simulink model "exercise03_simulation_model_solution_part1"  (R2025b)
settings: Solver=ode45  StartTime=0.0  StopTime=10  FixedStep=1e-5  MaxStep=1e-3  RelTol=1e-4  EnableMultiTasking=on
PreLoadFcn:
  | exercise03_simulation_parameters
values from neighbouring files (symbols this model uses):
  g = 9.81    [exercise03_solution_compute_LQR_outer_loop_controller.m]
undefined symbols (not defined in the file or in its folder): cmd_2_newtons_conversion_linear_coefficient, cmd_2_newtons_conversion_quadratic_coefficient, cmd_max, cmd_min, DiscIntNeverNeededParam, K_lqr, measurement_noise, nrotor_initial_conditions, nrotor_vehicle, pid_x, pid_y, pid_z, reference, sample_time, sigbuilder_block
libraries: simulink x3
(part 1 of 2)
settings Model: Creator=kimal and jseitz  LastModifiedBy=resjoehr
settings SolverCC: ZeroCrossControl=DisableAll  AlgebraicLoopSolver=TrustRegion  AutoInsertRateTranBlk=on
settings DataIOCC: LimitDataPoints=on  SaveFormat=Array  ReturnWorkspaceOutputs=off
settings OptimizationCC: LifeSpan=inf
settings DebuggingCC: SolverPrmCheckMsg=warning  UnconnectedInputMsg=warning  UnconnectedOutputMsg=warning  UnconnectedLineMsg=warning  SFUnexpectedBacktrackingDiag=warning  SFNoUnconditionalDefaultTransitionDiag=warning  SFExecutionAtInitializationDiag=none  ArithmeticOperatorsInVariantConditions=warning
settings HardwareCC: ProdBitPerPointer=32.0  ProdBitPerSizeT=32.0  ProdBitPerPtrDiffT=32.0  ProdLargestAtomicFloat=None  ProdIntDivRoundTo=Undefined  ProdEndianess=Unspecified  ProdWordSize=32.0  ProdHWDeviceType=32-bit Generic
settings ModelReferenceCC: EnableRefExpFcnMdlSchedulingChecks=on  PropagateSignalLabelsOutOfModel=off
settings SFSimCC: SimUseLocalCustomCode=off  CustomCodeUndefinedFunction=UseInterfaceOnly
settings RTWCC: RTWUseLocalCustomCode=off  GPUComputeCapability=3.5
settings CodeAppCC: StateflowObjectComments=on
settings GRTTargetCC: TargetLangStandard=C89/C90 (ANSI)
settings ConfigComp: CovMetricSettings=dw  CovSaveCumulativeToWorkspaceVar=on  CovSaveSingleToWorkspaceVar=on  CovExternalEMLEnable=off  CovSFcnEnable=off
settings SimscapeCC: SimscapeNormalizeSystem=off
settings ConfigurationSet: Description=SimMechanics 2G

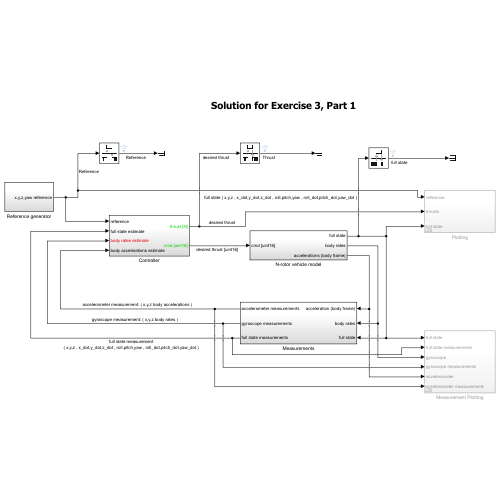
[thumbnail: Simulink's stored preview of the top-level diagram]
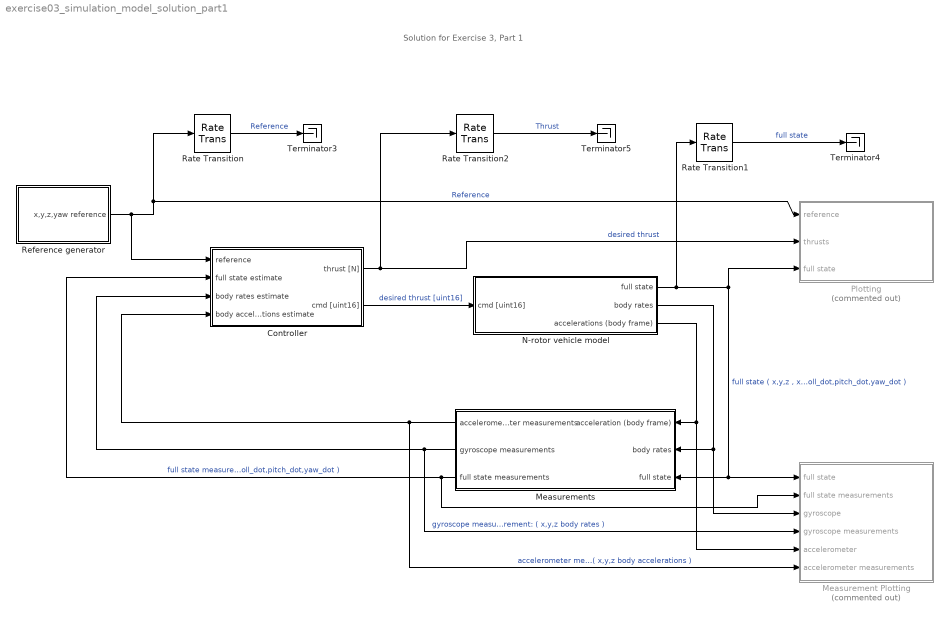
== system exercise03_simulation_model_solution_part1 ==
  note: Solution for Exercise 3, Part 1
  Controller : Subsystem
  Measurement Plotting : Subsystem  Commented=on
  Measurements : Subsystem
  N-rotor vehicle model : Subsystem
  Plotting : Subsystem  Commented=on
  Rate Transition : RateTransition  OutPortSampleTime=0.05
  Rate Transition1 : RateTransition  OutPortSampleTime=0.05
  Rate Transition2 : RateTransition  OutPortSampleTime=0.05
  Reference generator : Subsystem
  Terminator3 : Terminator
  Terminator4 : Terminator
  Terminator5 : Terminator
  wires:
  N-rotor vehicle model/2(body rates) -> Measurement Plotting/3(gyroscope), Measurements/2(body rates)
  N-rotor vehicle model/3(accelerations (body frame)) -> Measurement Plotting/5(accelerometer), Measurements/1(acceleration (body frame))
  Measurements/3(full state measurements) -> Controller/2(full state estimate), Measurement Plotting/2(full state measurements)  "full state measurement ( x,y,z , x_dot,y_dot,z_dot , roll,pitch,yaw , roll_dot,pitch_dot,yaw_dot )"
  Measurements/1(accelerometer measurements) -> Controller/4(body accelerations estimate), Measurement Plotting/6(accelerometer measurements)  "accelerometer measurement: ( x,y,z body accelerations )"
  Measurements/2(gyroscope measurements) -> Controller/3(body rates estimate), Measurement Plotting/4(gyroscope measurements)  "gyroscope measurement: ( x,y,z body rates )"
  Controller/2(cmd [uint16]) -> N-rotor vehicle model/1(cmd [uint16])  "desired thrust [uint16]"
  Reference generator/1(x,y,z,yaw reference) -> Controller/1(reference), Rate Transition/1, Plotting/1(reference)  "Reference"
  Rate Transition2/1 -> Terminator5/1  "Thrust"
  Rate Transition1/1 -> Terminator4/1  "full state"
  Controller/1(thrust [N]) -> Rate Transition2/1, Plotting/2(thrusts)  "desired thrust"
  Rate Transition/1 -> Terminator3/1  "Reference"
  N-rotor vehicle model/1(full state) -> Rate Transition1/1, Measurement Plotting/1(full state), Measurements/3(full state), Plotting/3(full state)  "full state ( x,y,z , x_dot,y_dot,z_dot , roll,pitch,yaw , roll_dot,pitch_dot,yaw_dot )"

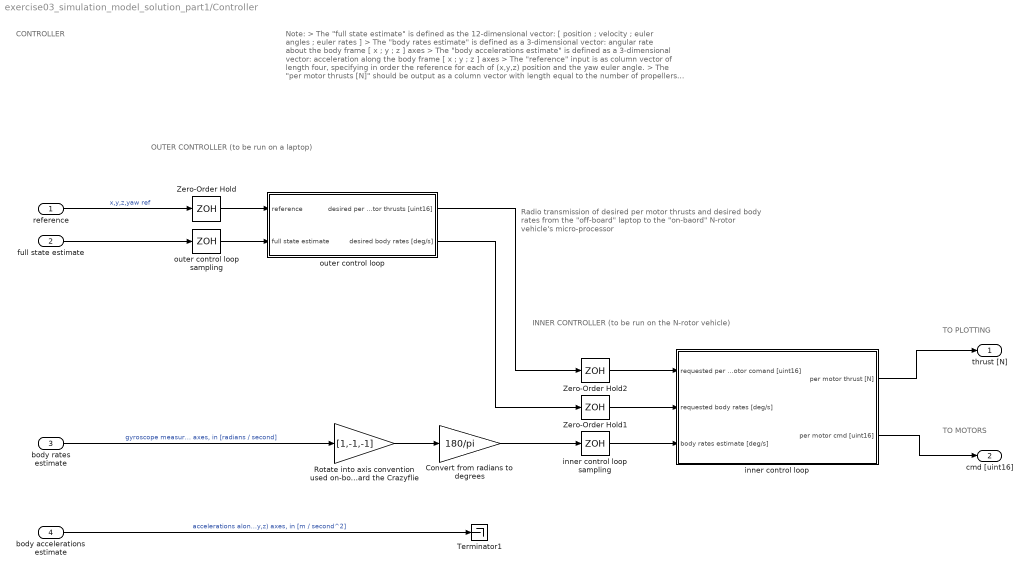
== system exercise03_simulation_model_solution_part1/Controller ==
  note: CONTROLLER
  note: Note:
      | > The "full state estimate" is defined as the 12-dimensional vector: [ position ; velocity ; euler angles ; euler rates ]
      | > The "body rates estimate" is defined as a 3-dimensional vector: angular rate about the body frame [ x ; y ; z ] axes
      | > The "body accelerations estimate" is defined as a 3-dimensional vector: acceleration along the body frame [ x ; y ; z ] axes
      | > The "reference" input is as column vector of length four, specifying in order the reference for each of (x,y,z) position and the yaw euler angle.
      | > The "per motor thrusts [N]" should be output as a column vector with length equal to the number of propellers on the vehicle, i.e., with length equal to N
      | > The "per motor cmd [uint16]" should be output as a column vector with length equal to the number of propellers on the vehicle, i.e., with length equal to N
  note: TO PLOTTING
  note: TO MOTORS
  note: Radio transmission of desired
      | per motor thrusts and desired
      | body rates from the "off-board"
      | laptop to the "on-baord" N-rotor
      | vehicle's micro-processor
  note: OUTER CONTROLLER (to be run on a laptop)
  note: INNER CONTROLLER (to be run on the N-rotor vehicle)
  reference : Inport
  full state estimate : Inport  Port=2
  body rates estimate : Inport  Port=3
  body accelerations estimate : Inport  Port=4
  Convert from radians to degrees : Gain  Gain=180/pi
  Rotate into axis convention used on-board the Crazyflie : Gain  Gain=[1,-1,-1]
  Terminator1 : Terminator
  Zero-Order Hold : ZeroOrderHold  SampleTime=sample_time.controller_outer
  Zero-Order Hold1 : ZeroOrderHold  SampleTime=sample_time.controller_inner
  Zero-Order Hold2 : ZeroOrderHold  SampleTime=sample_time.controller_inner
  inner control loop sampling : ZeroOrderHold  SampleTime=sample_time.controller_inner
  inner control loop : Subsystem
  outer control loop sampling : ZeroOrderHold  SampleTime=sample_time.controller_outer
  outer control loop : Subsystem
  thrust [N] : Outport  VectorParamsAs1DForOutWhenUnconnected=off
  cmd [uint16] : Outport  Port=2  VectorParamsAs1DForOutWhenUnconnected=off
  wires:
  body accelerations estimate/1 -> Terminator1/1  "accelerations along the body frame (x,y,z) axes, in [m / second^2]"
  body rates estimate/1 -> Rotate into axis convention used on-board the Crazyflie/1  "gyroscope measurement: angular rates about the body frame (x,y,z) axes, in [radians / second]"
  inner control loop/1(per motor thrust [N]) -> thrust [N]/1
  reference/1 -> Zero-Order Hold/1  "x,y,z,yaw ref"
  inner control loop/2(per motor cmd [uint16]) -> cmd [uint16]/1
  outer control loop sampling/1 -> outer control loop/2(full state estimate)
  full state estimate/1 -> outer control loop sampling/1
  outer control loop/2(desired body rates [deg/s]) -> Zero-Order Hold1/1
  Rotate into axis convention used on-board the Crazyflie/1 -> Convert from radians to degrees/1
  outer control loop/1(desired per motor thrusts [uint16]) -> Zero-Order Hold2/1
  Convert from radians to degrees/1 -> inner control loop sampling/1
  Zero-Order Hold1/1 -> inner control loop/2(requested body rates [deg/s])
  Zero-Order Hold/1 -> outer control loop/1(reference)
  Zero-Order Hold2/1 -> inner control loop/1(requested per motor comand [uint16])
  inner control loop sampling/1 -> inner control loop/3(body rates estimate [deg/s])

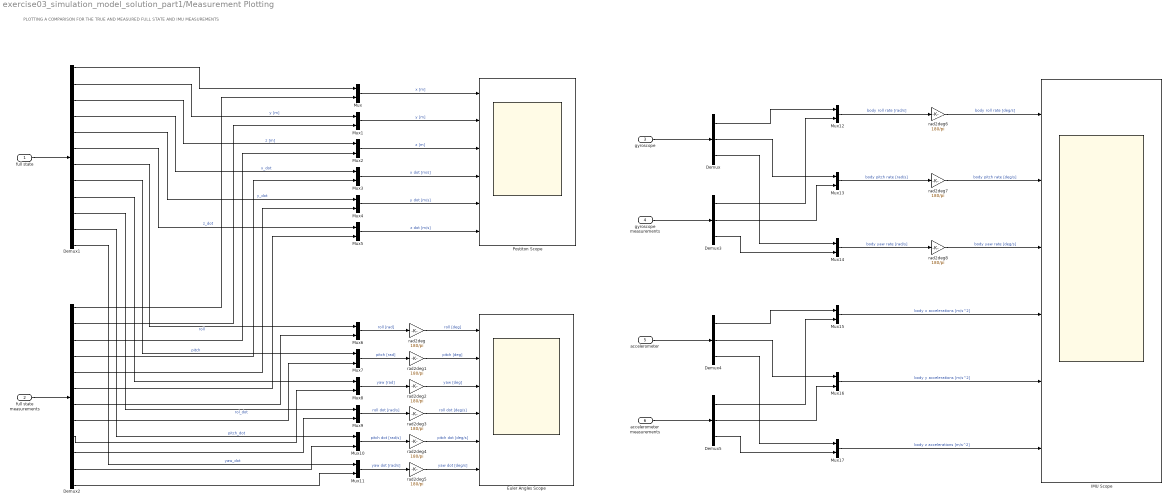
== system exercise03_simulation_model_solution_part1/Measurement Plotting ==
  note: PLOTTING A COMPARISON FOR THE TRUE AND MEASURED FULL STATE AND IMU MEASUREMENTS
  full state : Inport
  full state measurements : Inport  Port=2
  gyroscope : Inport  Port=3
  gyroscope measurements : Inport  Port=4
  accelerometer : Inport  Port=5
  accelerometer measurements : Inport  Port=6
  Demux{,3..5} (4 alike) : Demux  Outputs=3
  Demux1 : Demux  Outputs=12
  Demux2 : Demux  Outputs=12
  Euler Angles Scope : Scope  NumInputPorts=6
      settings: TimeSpan=10  ActiveDisplayYMinimum=-7.01847  ActiveDisplayYMaximum=5.9111  DataLoggingSaveFormat=Array
  IMU Scope : Scope  NumInputPorts=6
      settings: TimeSpan=10  ActiveDisplayYMinimum=-766.14622  ActiveDisplayYMaximum=735.9979  DataLoggingSaveFormat=Array
  Mux{,1..17} (18 alike) : Mux  Inputs=2
  Postiton Scope : Scope  NumInputPorts=6
      settings: TimeSpan=10  ActiveDisplayYMinimum=-0.0967  ActiveDisplayYMaximum=0.63434  DataLoggingSaveFormat=Array
  rad2deg{,1..8} (9 alike) : Gain  Gain=180/pi
  wires:
  full state/1 -> Demux1/1
  full state measurements/1 -> Demux2/1
  Mux/1 -> Postiton Scope/1  "x [m]"
  Mux1/1 -> Postiton Scope/2  "y [m]"
  Mux2/1 -> Postiton Scope/3  "z [m]"
  Mux3/1 -> Postiton Scope/4  "x dot [m/s]"
  Mux4/1 -> Postiton Scope/5  "y dot [m/s]"
  Mux5/1 -> Postiton Scope/6  "z dot [m/s]"
  Mux6/1 -> rad2deg/1  "roll [rad]"
  Mux7/1 -> rad2deg1/1  "pitch [rad]"
  Mux8/1 -> rad2deg2/1  "yaw [rad]"
  Mux9/1 -> rad2deg3/1  "roll dot [rad/s]"
  Mux10/1 -> rad2deg4/1  "pitch dot [rad/s]"
  Mux11/1 -> rad2deg5/1  "yaw dot [rad/s]"
  rad2deg/1 -> Euler Angles Scope/1  "roll [deg]"
  rad2deg2/1 -> Euler Angles Scope/3  "yaw [deg]"
  rad2deg1/1 -> Euler Angles Scope/2  "pitch [deg]"
  rad2deg3/1 -> Euler Angles Scope/4  "roll dot [deg/s]"
  rad2deg4/1 -> Euler Angles Scope/5  "pitch dot [deg/s]"
  rad2deg5/1 -> Euler Angles Scope/6  "yaw dot [deg/s]"
  Demux1/1 -> Mux/1
  Demux2/1 -> Mux/2
  Demux1/2 -> Mux1/1  "y [m]"
  Demux1/3 -> Mux2/1  "z [m]"
  Demux2/2 -> Mux1/2
  Demux2/3 -> Mux2/2
  Demux1/4 -> Mux3/1  "x_dot"
  Demux1/5 -> Mux4/1  "y_dot"
  Demux1/6 -> Mux5/1  "z_dot"
  Demux1/12 -> Mux11/1  "yaw_dot"
  Demux1/11 -> Mux10/1  "pitch_dot"
  Demux1/10 -> Mux9/1  "rol_dot"
  Demux1/9 -> Mux8/1
  Demux1/8 -> Mux7/1  "pitch"
  Demux1/7 -> Mux6/1  "roll"
  Demux2/4 -> Mux3/2
  Demux2/5 -> Mux4/2
  Demux2/6 -> Mux5/2
  Demux2/7 -> Mux6/2
  Demux2/8 -> Mux7/2
  Demux2/9 -> Mux8/2
  Demux2/10 -> Mux9/2
  Demux2/11 -> Mux10/2
  Demux2/12 -> Mux11/2
  gyroscope measurements/1 -> Demux3/1
  gyroscope/1 -> Demux/1
  Mux12/1 -> rad2deg6/1  "body roll rate [rad/s]"
  rad2deg6/1 -> IMU Scope/1  "body roll rate [deg/s]"
  Mux13/1 -> rad2deg7/1  "body pitch rate [rad/s]"
  rad2deg7/1 -> IMU Scope/2  "body pitch rate [deg/s]"
  Mux14/1 -> rad2deg8/1  "body yaw rate [rad/s]"
  rad2deg8/1 -> IMU Scope/3  "body yaw rate [deg/s]"
  Demux/1 -> Mux12/1
  Demux/2 -> Mux13/1
  Demux/3 -> Mux14/1
  Demux3/3 -> Mux14/2
  Demux3/2 -> Mux13/2
  Demux3/1 -> Mux12/2
  accelerometer measurements/1 -> Demux5/1
  accelerometer/1 -> Demux4/1
  Mux15/1 -> IMU Scope/4  "body x accelerations [m/s^2]"
  Mux16/1 -> IMU Scope/5  "body y accelerations [m/s^2]"
  Mux17/1 -> IMU Scope/6  "body z accelerations [m/s^2]"
  Demux4/1 -> Mux15/1
  Demux4/2 -> Mux16/1
  Demux4/3 -> Mux17/1
  Demux5/3 -> Mux17/2
  Demux5/2 -> Mux16/2
  Demux5/1 -> Mux15/2

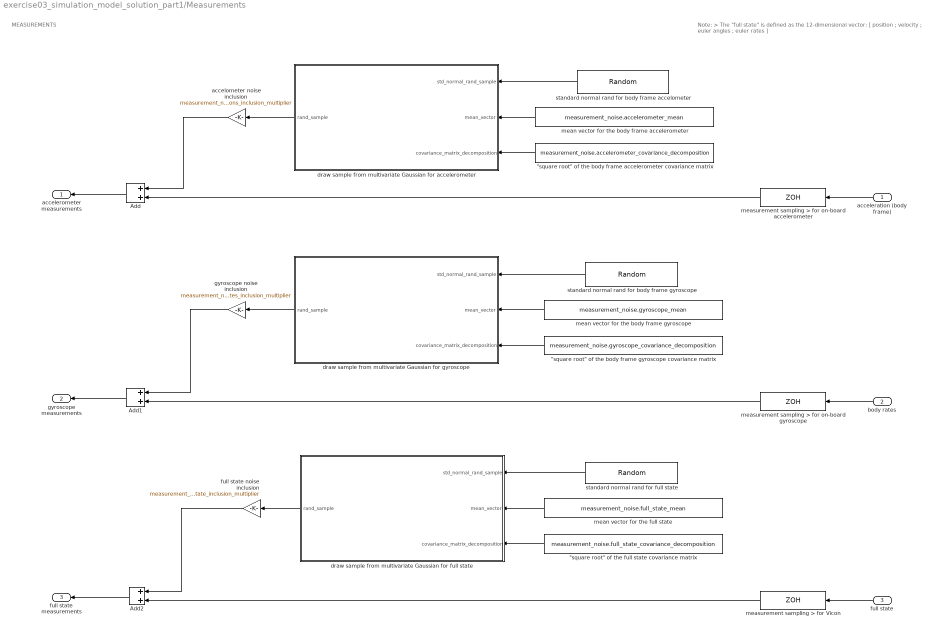
== system exercise03_simulation_model_solution_part1/Measurements ==
  note: Note:
      | > The "full state" is defined as the 12-dimensional vector:
      | [ position ; velocity ; euler angles ; euler rates ]
  note: MEASUREMENTS
  acceleration (body frame) : Inport
  body rates : Inport  Port=2
  full state : Inport  Port=3
  "\"square root\" of the body frame accelerometer covariance matrix" : Constant  Value=measurement_noise.accelerometer_covariance_decomposition
  "\"square root\" of the body frame gyroscope covariance matrix" : Constant  Value=measurement_noise.gyroscope_covariance_decomposition
  "\"square root\" of the full state covariance matrix" : Constant  Value=measurement_noise.full_state_covariance_decomposition
  Add : Sum
  Add1 : Sum
  Add2 : Sum
  accelometer noise inclusion : Gain  Gain=measurement_noise.body_accelerations_inclusion_multiplier
  draw sample from multivariate Gaussian for accelerometer : MATLAB Function  TreatAsAtomicUnit=on
  draw sample from multivariate Gaussian for full state : MATLAB Function  TreatAsAtomicUnit=on
  draw sample from multivariate Gaussian for gyroscope : MATLAB Function  TreatAsAtomicUnit=on
  full state noise inclusion : Gain  Gain=measurement_noise.full_state_inclusion_multiplier
  gyroscope noise inclusion : Gain  Gain=measurement_noise.body_rates_inclusion_multiplier
  mean vector for the body frame accelerometer : Constant  Value=measurement_noise.accelerometer_mean
  mean vector for the body frame gyroscope : Constant  Value=measurement_noise.gyroscope_mean
  mean vector for the full state : Constant  Value=measurement_noise.full_state_mean
  measurement sampling > for Vicon : ZeroOrderHold  SampleTime=sample_time.measurements_full_state
  measurement sampling > for on-board accelerometer : ZeroOrderHold  SampleTime=sample_time.measurements_body_accelerations
  measurement sampling > for on-board gyroscope : ZeroOrderHold  SampleTime=sample_time.measurements_body_rates
  standard normal rand for body frame accelometer : RandomNumber  Mean=measurement_noise.accelerometer_mean  Variance=measurement_noise.accelerometer_var  Seed=measurement_noise.accelerometer_seed  SampleTime=sample_time.measurements_body_accelerations  VectorParams1D=off
  standard normal rand for body frame gyroscope : RandomNumber  Mean=measurement_noise.gyroscope_mean  Variance=measurement_noise.gyroscope_var  Seed=measurement_noise.gyroscope_seed  SampleTime=sample_time.measurements_body_rates  VectorParams1D=off
  standard normal rand for full state : RandomNumber  Mean=zeros(12,1)  Variance=ones(12,1)  Seed=measurement_noise.full_state_seed  SampleTime=sample_time.measurements_full_state  VectorParams1D=off
  accelerometer measurements : Outport  VectorParamsAs1DForOutWhenUnconnected=off
  gyroscope measurements : Outport  Port=2  VectorParamsAs1DForOutWhenUnconnected=off
  full state measurements : Outport  Port=3  VectorParamsAs1DForOutWhenUnconnected=off
  wires:
  full state/1 -> measurement sampling > for Vicon/1
  acceleration (body frame)/1 -> measurement sampling > for on-board accelerometer/1
  body rates/1 -> measurement sampling > for on-board gyroscope/1
  measurement sampling > for Vicon/1 -> Add2/2
  "\"square root\" of the full state covariance matrix"/1 -> draw sample from multivariate Gaussian for full state/3(covariance_matrix_decomposition)
  mean vector for the full state/1 -> draw sample from multivariate Gaussian for full state/2(mean_vector)
  mean vector for the body frame gyroscope/1 -> draw sample from multivariate Gaussian for gyroscope/2(mean_vector)
  gyroscope noise inclusion/1 -> Add1/1
  measurement sampling > for on-board accelerometer/1 -> Add/2
  mean vector for the body frame accelerometer/1 -> draw sample from multivariate Gaussian for accelerometer/2(mean_vector)
  draw sample from multivariate Gaussian for accelerometer/1(rand_sample) -> accelometer noise inclusion/1
  draw sample from multivariate Gaussian for gyroscope/1(rand_sample) -> gyroscope noise inclusion/1
  standard normal rand for full state/1 -> draw sample from multivariate Gaussian for full state/1(std_normal_rand_sample)
  "\"square root\" of the body frame gyroscope covariance matrix"/1 -> draw sample from multivariate Gaussian for gyroscope/3(covariance_matrix_decomposition)
  accelometer noise inclusion/1 -> Add/1
  draw sample from multivariate Gaussian for full state/1(rand_sample) -> full state noise inclusion/1
  full state noise inclusion/1 -> Add2/1
  measurement sampling > for on-board gyroscope/1 -> Add1/2
  standard normal rand for body frame gyroscope/1 -> draw sample from multivariate Gaussian for gyroscope/1(std_normal_rand_sample)
  standard normal rand for body frame accelometer/1 -> draw sample from multivariate Gaussian for accelerometer/1(std_normal_rand_sample)
  Add2/1 -> full state measurements/1
  "\"square root\" of the body frame accelerometer covariance matrix"/1 -> draw sample from multivariate Gaussian for accelerometer/3(covariance_matrix_decomposition)
  Add/1 -> accelerometer measurements/1
  Add1/1 -> gyroscope measurements/1

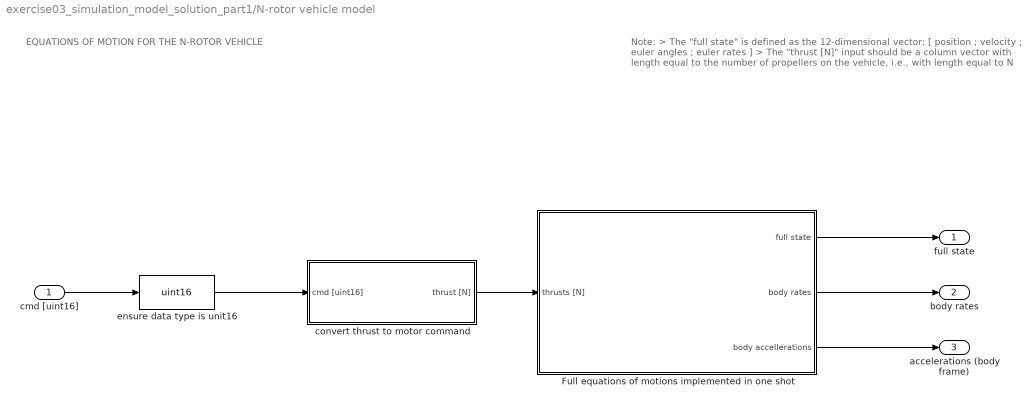
== system exercise03_simulation_model_solution_part1/N-rotor vehicle model ==
  note: Note:
      | > The "full state" is defined as the 12-dimensional vector:
      | [ position ; velocity ; euler angles ; euler rates ]
      | > The "thrust [N]" input should be a column vector with
      | length equal to the number of propellers on the vehicle,
      | i.e., with length equal to N
  note: EQUATIONS OF MOTION FOR THE N-ROTOR VEHICLE
  cmd [uint16] : Inport
  Full equations of motions implemented in one shot : Subsystem
  convert thrust to motor command : Subsystem
  ensure data type is unit16 : DataTypeConversion  OutDataTypeStr=uint16  SaturateOnIntegerOverflow=off  RndMeth=Floor
  full state : Outport  VectorParamsAs1DForOutWhenUnconnected=off
  body rates : Outport  Port=2  VectorParamsAs1DForOutWhenUnconnected=off
  accelerations (body frame) : Outport  Port=3  VectorParamsAs1DForOutWhenUnconnected=off
  wires:
  cmd [uint16]/1 -> ensure data type is unit16/1
  Full equations of motions implemented in one shot/1(full state) -> full state/1
  Full equations of motions implemented in one shot/2(body rates) -> body rates/1
  Full equations of motions implemented in one shot/3(body accellerations) -> accelerations (body frame)/1
  convert thrust to motor command/1(thrust [N]) -> Full equations of motions implemented in one shot/1(thrusts [N])
  ensure data type is unit16/1 -> convert thrust to motor command/1(cmd [uint16])

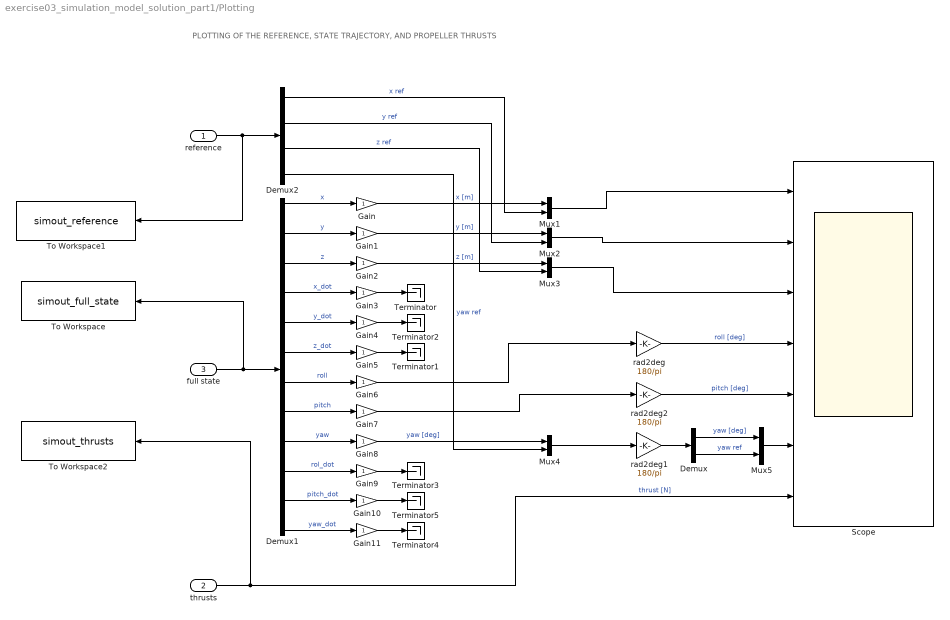
== system exercise03_simulation_model_solution_part1/Plotting ==
  note: PLOTTING OF THE REFERENCE, STATE TRAJECTORY, AND PROPELLER THRUSTS
  reference : Inport
  thrusts : Inport  Port=2
  full state : Inport  Port=3
  Demux : Demux  Outputs=2
  Demux1 : Demux  Outputs=12
  Demux2 : Demux
  Gain{,1..11} (12 alike) : Gain
  Mux{1..5} (5 alike) : Mux  Inputs=2
  Scope : Scope  NumInputPorts=7
      settings: TimeSpan=10  ActiveDisplayYMinimum=-1.3075  ActiveDisplayYMaximum=11.45582  DataLoggingSaveFormat=Array
  Terminator{,1..5} (6 alike) : Terminator
  To Workspace : ToWorkspace  VariableName=simout_full_state  SaveFormat=Timeseries  SampleTime=-1
  To Workspace1 : ToWorkspace  VariableName=simout_reference  SaveFormat=Timeseries  SampleTime=-1
  To Workspace2 : ToWorkspace  VariableName=simout_thrusts  SaveFormat=Timeseries  SampleTime=-1
  rad2deg : Gain  Gain=180/pi
  rad2deg1 : Gain  Gain=180/pi
  rad2deg2 : Gain  Gain=180/pi
  wires:
  Demux1/1 -> Gain/1  "x"
  Demux1/2 -> Gain1/1  "y"
  Demux1/6 -> Gain5/1  "z_dot"
  Gain7/1 -> rad2deg2/1
  Demux1/8 -> Gain7/1  "pitch"
  full state/1 -> To Workspace/1, Demux1/1
  Demux1/5 -> Gain4/1  "y_dot"
  Demux1/7 -> Gain6/1  "roll"
  Demux1/4 -> Gain3/1  "x_dot"
  Demux1/3 -> Gain2/1  "z"
  Gain6/1 -> rad2deg/1
  Demux1/9 -> Gain8/1  "yaw"
  Demux1/10 -> Gain9/1  "rol_dot"
  Demux1/11 -> Gain10/1  "pitch_dot"
  Demux1/12 -> Gain11/1  "yaw_dot"
  Gain9/1 -> Terminator3/1
  Gain10/1 -> Terminator5/1
  Gain11/1 -> Terminator4/1
  Gain3/1 -> Terminator/1
  Gain4/1 -> Terminator2/1
  Gain5/1 -> Terminator1/1
  thrusts/1 -> To Workspace2/1, Scope/7  "thrust [N]"
  reference/1 -> To Workspace1/1, Demux2/1
  Mux1/1 -> Scope/1
  Mux2/1 -> Scope/2
  Gain/1 -> Mux1/1  "x [m]"
  Demux2/1 -> Mux1/2  "x ref"
  Gain1/1 -> Mux2/1  "y [m]"
  Demux2/2 -> Mux2/2  "y ref"
  Mux3/1 -> Scope/3
  Gain2/1 -> Mux3/1  "z [m]"
  Demux2/3 -> Mux3/2  "z ref"
  Mux4/1 -> rad2deg1/1
  Gain8/1 -> Mux4/1  "yaw [deg]"
  Demux2/4 -> Mux4/2  "yaw ref"
  rad2deg/1 -> Scope/4  "roll [deg]"
  rad2deg2/1 -> Scope/5  "pitch [deg]"
  Demux/1 -> Mux5/1  "yaw [deg]"
  Demux/2 -> Mux5/2  "yaw ref"
  rad2deg1/1 -> Demux/1
  Mux5/1 -> Scope/6

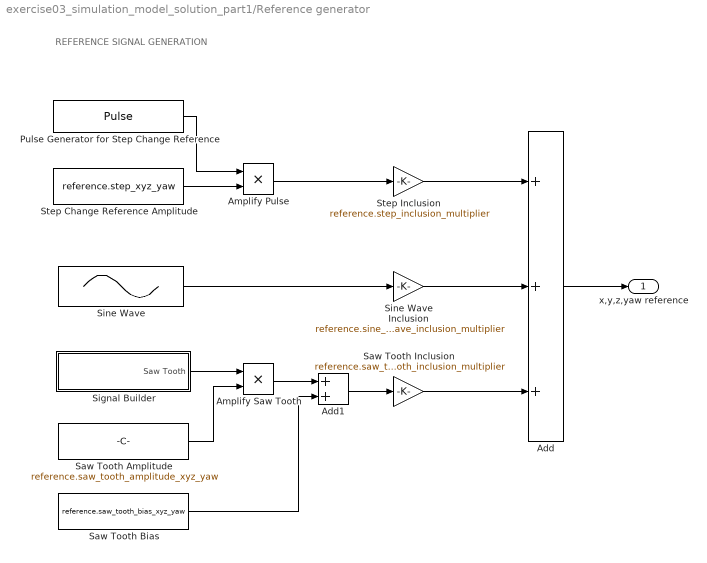
== system exercise03_simulation_model_solution_part1/Reference generator ==
  note: REFERENCE SIGNAL GENERATION
  Add : Sum  Inputs=+++
  Add1 : Sum
  Amplify Pulse : Product
  Amplify Saw Tooth : Product
  Pulse Generator for Step Change Reference : DiscretePulseGenerator  PulseType=Time based  Period=reference.step_period*2  PulseWidth=50
  Saw Tooth Amplitude : Constant  Value=reference.saw_tooth_amplitude_xyz_yaw
  Saw Tooth Bias : Constant  Value=reference.saw_tooth_bias_xyz_yaw
  Saw Tooth Inclusion : Gain  Gain=reference.saw_tooth_inclusion_multiplier
  Signal Builder : Subsystem  Tag=STV Subsys  LoadFcn=sigbuilder_block('load');  StartFcn=sigbuilder_block('start');  StopFcn=sigbuilder_block('stop');  ClipboardFcn=sigbuilder_block('clipboard');  mask(Sigbuilder block){tuvar=[0:10]}
      mask help: Simulink:masks:SigbuilderBlock_MD
      mask init:
      | if ~strcmp(get_param(bdroot(gcbh),'SimulationStatus'),'stopped') tuvar = sigbuilder_block('maskInit'); end
      settings: CopyFcn=sigbuilder_block('copy');  DeleteFcn=sigbuilder_block('delete');  ModelCloseFcn=sigbuilder_block('modelClose');  PreSaveFcn=sigbuilder_block('preSave');  PauseFcn=sigbuilder_block('pause');  ContinueFcn=sigbuilder_block('continue');  NameChangeFcn=sigbuilder_block('namechange');  OpenFcn=sigbuilder_block('open',[-1646.25 158.25 895.5 539.25 ]);  CloseFcn=sigbuilder_block('close');
      mask Display: plot(0, 0, 100, 100,[2, 2, 32, 32, 2], [68, 8, 8, 68, 68],[32, 2], [38, 38], [32, 19, 2],[53, 60, 44], [32, 17, 17, 2],[16, 16, 31, 31]);txt = getActiveGroup(gcbh);text(2, 100, txt,'verticalAlignment', 'top');
  Sine Wave : Sin  Amplitude=reference.sine_amplitude_xyz_yaw  Bias=reference.sine_bias_xyz_yaw  Frequency=2*pi()/reference.sine_period  SampleTime=0
  Sine Wave Inclusion : Gain  Gain=reference.sine_wave_inclusion_multiplier
  Step Change Reference Amplitude : Constant  Value=reference.step_xyz_yaw
  Step Inclusion : Gain  Gain=reference.step_inclusion_multiplier
  x,y,z,yaw reference : Outport  VectorParamsAs1DForOutWhenUnconnected=off
  wires:
  Step Change Reference Amplitude/1 -> Amplify Pulse/2
  Pulse Generator for Step Change Reference/1 -> Amplify Pulse/1
  Sine Wave/1 -> Sine Wave Inclusion/1
  Add/1 -> x,y,z,yaw reference/1
  Step Inclusion/1 -> Add/1
  Sine Wave Inclusion/1 -> Add/2
  Amplify Pulse/1 -> Step Inclusion/1
  Saw Tooth Inclusion/1 -> Add/3
  Signal Builder/1(Saw Tooth) -> Amplify Saw Tooth/1
  Saw Tooth Amplitude/1 -> Amplify Saw Tooth/2
  Amplify Saw Tooth/1 -> Add1/1
  Add1/1 -> Saw Tooth Inclusion/1
  Saw Tooth Bias/1 -> Add1/2

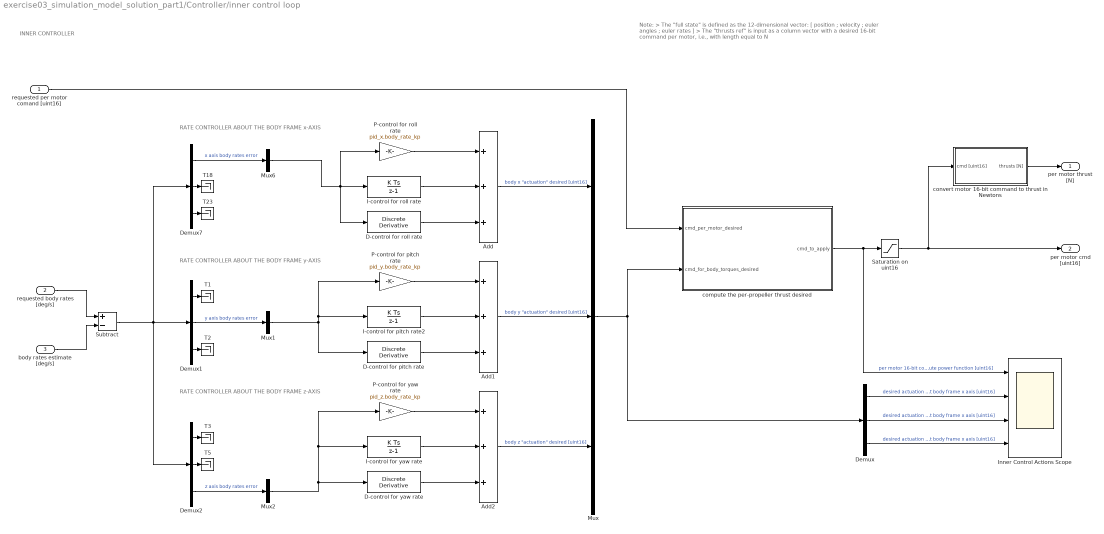
== system exercise03_simulation_model_solution_part1/Controller/inner control loop ==
  note: RATE CONTROLLER ABOUT THE BODY FRAME z-AXIS
  note: RATE CONTROLLER ABOUT THE BODY FRAME y-AXIS
  note: RATE CONTROLLER ABOUT THE BODY FRAME x-AXIS
  note: INNER CONTROLLER
  note: Note:
      | > The "full state" is defined as the 12-dimensional vector:
      | [ position ; velocity ; euler angles ; euler rates ]
      | > The "thrusts ref" is input as a column vector with a desired
      | 16-bit command per motor, i.e., with length equal to N
  requested per motor comand [uint16] : Inport
  requested body rates [deg/s] : Inport  Port=2
  body rates estimate [deg/s] : Inport  Port=3
  Add : Sum  Inputs=+++
  Add1 : Sum  Inputs=+++
  Add2 : Sum  Inputs=+++
  D-control for pitch rate : simulink/Discrete/Discrete Derivative  gainval=pid_y.body_rate_kd  ICPrevScaledInput=0.0  OutMin=[]  OutMax=[]  OutDataType=fixdt(1, 16)  OutScaling=2^-10  DoSatur=off
  D-control for roll rate : simulink/Discrete/Discrete Derivative  gainval=pid_x.body_rate_kd  ICPrevScaledInput=0.0  OutMin=[]  OutMax=[]  OutDataType=fixdt(1, 16)  OutScaling=2^-10  DoSatur=off
  D-control for yaw rate : simulink/Discrete/Discrete Derivative  gainval=pid_z.body_rate_kd  ICPrevScaledInput=0.0  OutMin=[]  OutMax=[]  OutDataType=fixdt(1, 16)  OutScaling=2^-10  DoSatur=off
  Demux{,1..2,7} (4 alike) : Demux  Outputs=3
  I-control for pitch rate2 : DiscreteIntegrator  gainval=pid_y.body_rate_ki  SampleTime=-1  LimitOutput=on  UpperSaturationLimit=pid_y.body_rate_integrator_limit  LowerSaturationLimit=-pid_y.body_rate_integrator_limit  ICPrevOutput=DiscIntNeverNeededParam  ICPrevScaledInput=DiscIntNeverNeededParam
  I-control for roll rate : DiscreteIntegrator  gainval=pid_x.body_rate_ki  SampleTime=-1  LimitOutput=on  UpperSaturationLimit=pid_x.body_rate_integrator_limit  LowerSaturationLimit=-pid_x.body_rate_integrator_limit  ICPrevOutput=DiscIntNeverNeededParam  ICPrevScaledInput=DiscIntNeverNeededParam
  I-control for yaw rate : DiscreteIntegrator  gainval=pid_z.body_rate_ki  SampleTime=-1  LimitOutput=on  UpperSaturationLimit=pid_x.body_rate_integrator_limit  LowerSaturationLimit=-pid_x.body_rate_integrator_limit  ICPrevOutput=DiscIntNeverNeededParam  ICPrevScaledInput=DiscIntNeverNeededParam
  Inner Control Actions Scope : Scope  NumInputPorts=4
      settings: ActiveDisplayYMinimum=36280.75  ActiveDisplayYMaximum=47683.25
  Mux : Mux  Inputs=3
  Mux1 : Mux  Inputs=1
  Mux2 : Mux  Inputs=1
  Mux6 : Mux  Inputs=1
  P-control for pitch rate : Gain  Gain=pid_y.body_rate_kp
  P-control for roll rate : Gain  Gain=pid_x.body_rate_kp
  P-control for yaw rate : Gain  Gain=pid_z.body_rate_kp
  Saturation on uint16 : Saturate  UpperLimit=cmd_max  LowerLimit=cmd_min  ZeroCross=off
  Subtract : Sum  Inputs=+-
  T{1..3,5,18,23} (6 alike) : Terminator
  compute the per-propeller thrust desired : MATLAB Function  TreatAsAtomicUnit=on
  convert motor 16-bit command to thrust in Newtons : Subsystem
  per motor thrust [N] : Outport  VectorParamsAs1DForOutWhenUnconnected=off
  per motor cmd [uint16] : Outport  Port=2  VectorParamsAs1DForOutWhenUnconnected=off
  wires:
  compute the per-propeller thrust desired/1(cmd_to_apply) -> Inner Control Actions Scope/1, Saturation on uint16/1  "per motor 16-bit command after distribute power function [uint16]"
  body rates estimate [deg/s]/1 -> Subtract/2
  requested per motor comand [uint16]/1 -> compute the per-propeller thrust desired/1(cmd_per_motor_desired)
  requested body rates [deg/s]/1 -> Subtract/1
  Add/1 -> Mux/1  "body x \"actuation\" desired [uint16]"
  Add1/1 -> Mux/2  "body y \"actuation\" desired [uint16]"
  Add2/1 -> Mux/3  "body z \"actuation\" desired [uint16]"
  Subtract/1 -> Demux2/1, Demux1/1, Demux7/1
  Mux/1 -> Demux/1, compute the per-propeller thrust desired/2(cmd_for_body_torques_desired)
  Saturation on uint16/1 -> per motor cmd [uint16]/1, convert motor 16-bit command to thrust in Newtons/1(cmd [uint16])
  Demux/1 -> Inner Control Actions Scope/2  "desired actuation about body frame x axis [uint16]"
  Demux/2 -> Inner Control Actions Scope/3  "desired actuation about body frame x axis [uint16]"
  Demux/3 -> Inner Control Actions Scope/4  "desired actuation about body frame x axis [uint16]"
  Demux7/2 -> T18/1
  Mux6/1 -> P-control for roll rate/1, I-control for roll rate/1, D-control for roll rate/1
  Demux7/3 -> T23/1
  Demux7/1 -> Mux6/1  "x axis body rates error"
  Demux1/2 -> Mux1/1  "y axis body rates error"
  Demux1/3 -> T2/1
  Demux1/1 -> T1/1
  Demux2/3 -> Mux2/1  "z axis body rates error"
  Demux2/1 -> T3/1
  Mux2/1 -> I-control for yaw rate/1, P-control for yaw rate/1, D-control for yaw rate/1
  Demux2/2 -> T5/1
  convert motor 16-bit command to thrust in Newtons/1(thrusts [N]) -> per motor thrust [N]/1
  P-control for roll rate/1 -> Add/1
  I-control for roll rate/1 -> Add/2
  D-control for roll rate/1 -> Add/3
  P-control for pitch rate/1 -> Add1/1
  I-control for pitch rate2/1 -> Add1/2
  D-control for pitch rate/1 -> Add1/3
  Mux1/1 -> D-control for pitch rate/1, P-control for pitch rate/1, I-control for pitch rate2/1
  D-control for yaw rate/1 -> Add2/3
  P-control for yaw rate/1 -> Add2/1
  I-control for yaw rate/1 -> Add2/2

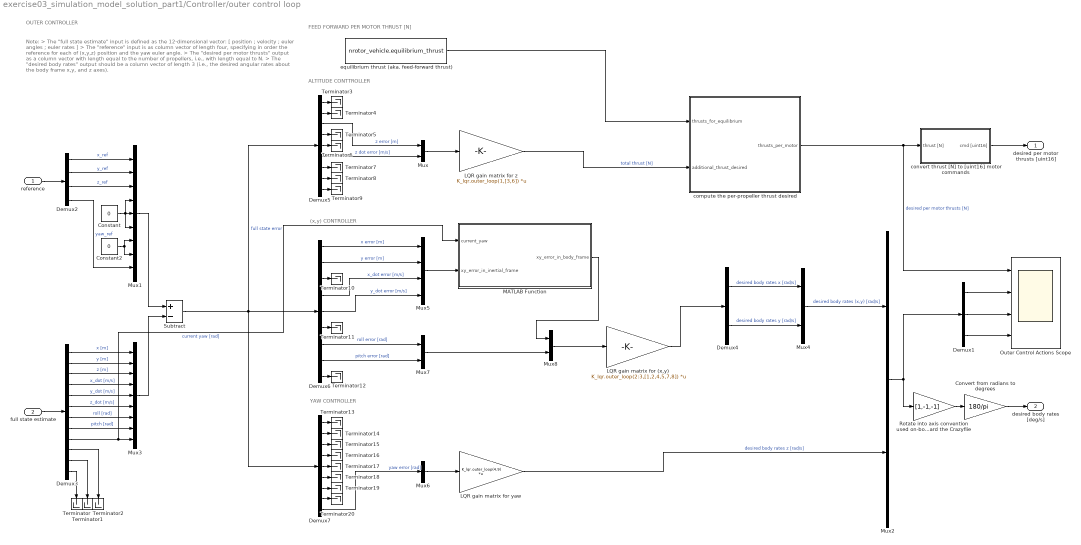
== system exercise03_simulation_model_solution_part1/Controller/outer control loop ==
  note: FEED FORWARD PER MOTOR THRUST [N]
  note: YAW CONTROLLER
  note: (x,y) CONTROLLER
  note: ALTITUDE CONTTROLLER
  note: OUTER CONTROLLER
  note: Note:
      | > The "full state estimate" input is defined as the 12-dimensional vector:
      | [ position ; velocity ; euler angles ; euler rates ]
      | > The "reference" input is as column vector of length four, specifying in
      | order the reference for each of (x,y,z) position and the yaw euler angle.
      | > The "desired per motor thrusts" output as a column vector with length
      | equal to the number of propellers, i.e., with length equal to N.
      | > The "desired body rates" output should be a column vector of length 3
      | (i.e., the desired angular rates about the body frame x,y, and z axes).
  reference : Inport
  full state estimate : Inport  Port=2
  Constant : Constant  Value=0
  Constant2 : Constant  Value=0
  Convert from radians to degrees : Gain  Gain=180/pi
  Demux1 : Demux  Outputs=3
  Demux2 : Demux
  Demux3 : Demux  Outputs=12
  Demux4 : Demux  Outputs=2
  Demux5 : Demux  Outputs=9
  Demux6 : Demux  Outputs=9
  Demux7 : Demux  Outputs=9
  LQR gain matrix for (x,y) : Gain  Gain=K_lqr.outer_loop(2:3,[1,2,4,5,7,8])  Multiplication=Matrix(K*u)
  LQR gain matrix for yaw : Gain  Gain=K_lqr.outer_loop(4,9)  Multiplication=Matrix(K*u)
  LQR gain matrix for z : Gain  Gain=K_lqr.outer_loop(1,[3,6])  Multiplication=Matrix(K*u)
  MATLAB Function : MATLAB Function  TreatAsAtomicUnit=on
  Mux{,2,4,7..8} (5 alike) : Mux  Inputs=2
  Mux1 : Mux  Inputs=9
  Mux3 : Mux  Inputs=9
  Mux5 : Mux
  Mux6 : Mux  Inputs=1
  Outer Control Actions Scope : Scope  NumInputPorts=4
      settings: ActiveDisplayYMinimum=0.06847  ActiveDisplayYMaximum=0.08971
  Rotate into axis convention used on-board the Crazyflie : Gain  Gain=[1,-1,-1]
  Subtract : Sum  Inputs=+-
  Terminator{,1..20} (21 alike) : Terminator
  compute the per-propeller thrust desired : MATLAB Function  TreatAsAtomicUnit=on
  convert thrust [N] to [uint16] motor commands : Subsystem
  equilibrium thrust (aka. feed-forward thrust) : Constant  Value=nrotor_vehicle.equilibrium_thrust
  desired per motor thrusts [uint16] : Outport  VectorParamsAs1DForOutWhenUnconnected=off
  desired body rates [deg/s] : Outport  Port=2  VectorParamsAs1DForOutWhenUnconnected=off
  wires:
  Mux1/1 -> Subtract/1
  reference/1 -> Demux2/1
  Demux2/1 -> Mux1/1  "x_ref"
  equilibrium thrust (aka. feed-forward thrust)/1 -> compute the per-propeller thrust desired/1(thrusts_for_equilibrium)
  Constant2/1 -> Mux1/8, Mux1/7
  Demux2/3 -> Mux1/3  "z_ref"
  Demux2/2 -> Mux1/2  "y_ref"
  Demux2/4 -> Mux1/9  "yaw_ref"
  Constant/1 -> Mux1/6, Mux1/4, Mux1/5
  LQR gain matrix for z/1 -> compute the per-propeller thrust desired/2(additional_thrust_desired)  "total thrust [N]"
  compute the per-propeller thrust desired/1(thrusts_per_motor) -> convert thrust [N] to [uint16] motor commands/1(thrust [N]), Outer Control Actions Scope/1  "desired per motor thrusts [N]"
  full state estimate/1 -> Demux3/1
  Demux3/1 -> Mux3/1  "x [m]"
  Demux3/2 -> Mux3/2  "y [m]"
  Demux3/3 -> Mux3/3  "z [m]"
  Demux3/4 -> Mux3/4  "x_dot [m/s]"
  Demux3/5 -> Mux3/5  "y_dot [m/s]"
  Demux3/7 -> Mux3/7  "roll [rad]"
  Demux3/6 -> Mux3/6  "z_dot [m/s]"
  Demux3/8 -> Mux3/8  "pitch [rad]"
  Demux3/9 -> MATLAB Function/1(current_yaw), Mux3/9  "current yaw [rad]"
  Demux3/10 -> Terminator2/1
  Demux3/11 -> Terminator1/1
  Demux3/12 -> Terminator/1
  Mux3/1 -> Subtract/2
  Demux1/3 -> Outer Control Actions Scope/4
  Demux1/2 -> Outer Control Actions Scope/3
  Demux1/1 -> Outer Control Actions Scope/2
  Subtract/1 -> Demux7/1, Demux5/1, Demux6/1  "full state error"
  LQR gain matrix for yaw/1 -> Mux2/2  "desired body rates z [rad/s]"
  LQR gain matrix for (x,y)/1 -> Demux4/1
  Demux4/2 -> Mux4/2  "desired body rates y [rad/s]"
  Demux4/1 -> Mux4/1  "desired body rates x [rad/s]"
  Mux4/1 -> Mux2/1  "desired body rates (x,y) [rad/s]"
  Demux5/3 -> Mux/1  "z error [m]"
  Demux5/6 -> Mux/2  "z dot error [m/s]"
  Demux5/1 -> Terminator3/1
  Demux5/2 -> Terminator4/1
  Demux5/4 -> Terminator5/1
  Demux5/5 -> Terminator6/1
  Demux5/7 -> Terminator7/1
  Demux5/8 -> Terminator8/1
  Demux5/9 -> Terminator9/1
  Mux/1 -> LQR gain matrix for z/1
  Demux6/1 -> Mux5/1  "x error [m]"
  Demux6/2 -> Mux5/2  "y error [m]"
  Demux6/4 -> Mux5/3  "x_dot error [m/s]"
  Demux6/5 -> Mux5/4  "y_dot error [m/s]"
  Demux6/7 -> Mux7/1  "roll error [rad]"
  Demux6/8 -> Mux7/2  "pitch error [rad]"
  Demux6/9 -> Terminator12/1
  Mux8/1 -> LQR gain matrix for (x,y)/1
  Demux6/6 -> Terminator11/1
  Demux6/3 -> Terminator10/1
  Demux7/1 -> Terminator13/1
  Demux7/2 -> Terminator14/1
  Demux7/4 -> Terminator16/1
  Demux7/5 -> Terminator17/1
  Demux7/7 -> Terminator19/1
  Demux7/8 -> Terminator20/1
  Demux7/9 -> Mux6/1  "yaw error [rad]"
  Mux6/1 -> LQR gain matrix for yaw/1
  Demux7/3 -> Terminator15/1
  Demux7/6 -> Terminator18/1
  Mux7/1 -> Mux8/2
  Mux5/1 -> MATLAB Function/2(xy_error_in_inertial_frame)
  MATLAB Function/1(xy_error_in_body_frame) -> Mux8/1
  convert thrust [N] to [uint16] motor commands/1(cmd [uint16]) -> desired per motor thrusts [uint16]/1
  Mux2/1 -> Rotate into axis convention used on-board the Crazyflie/1, Demux1/1
  Convert from radians to degrees/1 -> desired body rates [deg/s]/1
  Rotate into axis convention used on-board the Crazyflie/1 -> Convert from radians to degrees/1

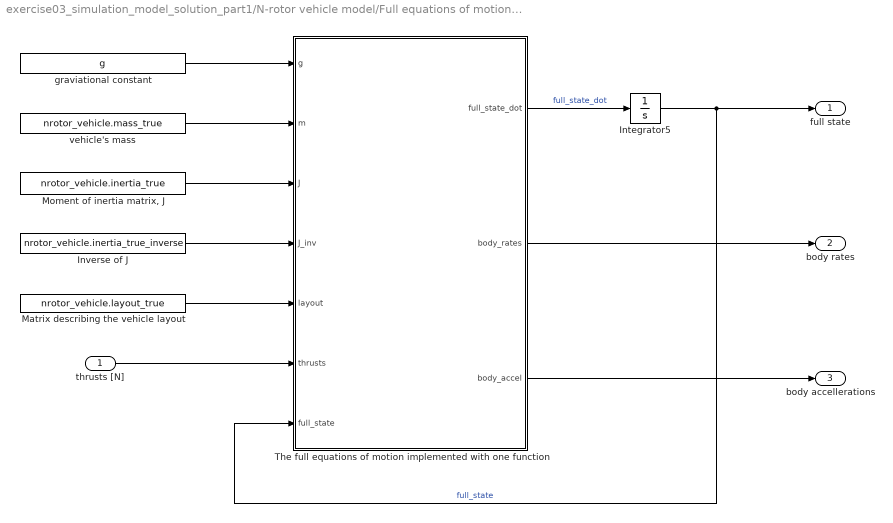
== system exercise03_simulation_model_solution_part1/N-rotor vehicle model/Full equations of motions implemented in one shot ==
  thrusts [N] : Inport
  Integrator5 : Integrator  InitialCondition=nrotor_initial_conditions
  Inverse of J : Constant  Value=nrotor_vehicle.inertia_true_inverse
  Matrix describing the vehicle layout : Constant  Value=nrotor_vehicle.layout_true
  "Moment of inertia matrix, J" : Constant  Value=nrotor_vehicle.inertia_true
  The full equations of motion implemented with one function : MATLAB Function  TreatAsAtomicUnit=on
  graviational constant : Constant  Value=g
  vehicle's mass : Constant  Value=nrotor_vehicle.mass_true
  full state : Outport  VectorParamsAs1DForOutWhenUnconnected=off
  body rates : Outport  Port=2  VectorParamsAs1DForOutWhenUnconnected=off
  body accellerations : Outport  Port=3  VectorParamsAs1DForOutWhenUnconnected=off
  wires:
  The full equations of motion implemented with one function/1(full_state_dot) -> Integrator5/1  "full_state_dot"
  Matrix describing the vehicle layout/1 -> The full equations of motion implemented with one function/5(layout)
  The full equations of motion implemented with one function/3(body_accel) -> body accellerations/1
  graviational constant/1 -> The full equations of motion implemented with one function/1(g)
  thrusts [N]/1 -> The full equations of motion implemented with one function/6(thrusts)
  The full equations of motion implemented with one function/2(body_rates) -> body rates/1
  Integrator5/1 -> full state/1, The full equations of motion implemented with one function/7(full_state)  "full_state"
  Inverse of J/1 -> The full equations of motion implemented with one function/4(J_inv)
  vehicle's mass/1 -> The full equations of motion implemented with one function/2(m)
  "Moment of inertia matrix, J"/1 -> The full equations of motion implemented with one function/3(J)

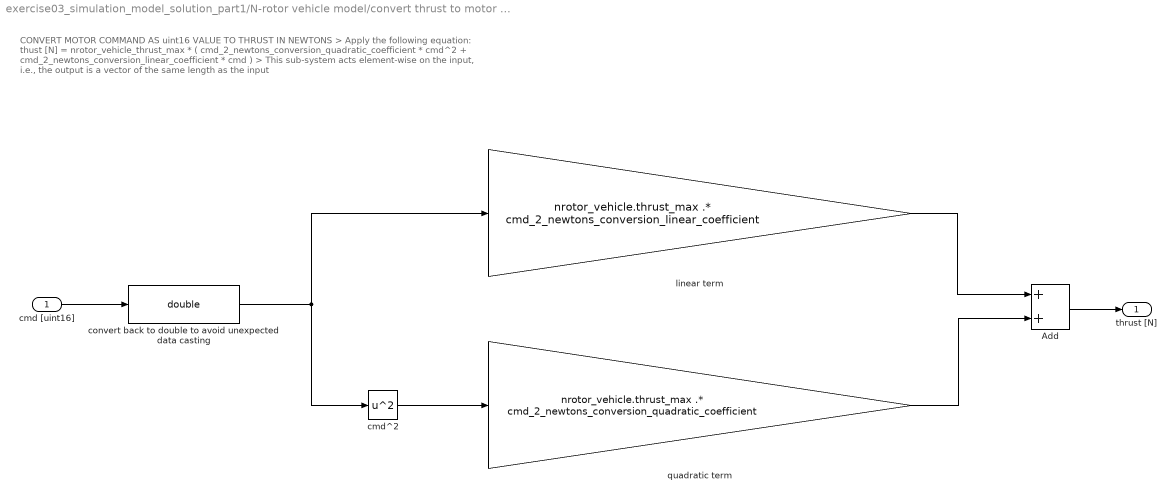
== system exercise03_simulation_model_solution_part1/N-rotor vehicle model/convert thrust to motor command ==
  note: CONVERT MOTOR COMMAND AS uint16 VALUE TO THRUST IN NEWTONS
      | > Apply the following equation:
      | thust [N] = nrotor_vehicle_thrust_max * ( cmd_2_newtons_conversion_quadratic_coefficient * cmd^2 + cmd_2_newtons_conversion_linear_coefficient * cmd )
      |
      | > This sub-system acts element-wise on the input, i.e., the output is a vector of the same length as the input
  cmd [uint16] : Inport
  Add : Sum
  cmd^2 : Math  Operator=square  SignedPower=on
  convert back to double to avoid unexpected data casting : DataTypeConversion  OutDataTypeStr=double  SaturateOnIntegerOverflow=off  RndMeth=Floor
  linear term : Gain  Gain=nrotor_vehicle.thrust_max .* cmd_2_newtons_conversion_linear_coefficient
  quadratic term : Gain  Gain=nrotor_vehicle.thrust_max .* cmd_2_newtons_conversion_quadratic_coefficient
  thrust [N] : Outport  VectorParamsAs1DForOutWhenUnconnected=off
  wires:
  cmd^2/1 -> quadratic term/1
  quadratic term/1 -> Add/2
  linear term/1 -> Add/1
  cmd [uint16]/1 -> convert back to double to avoid unexpected data casting/1
  Add/1 -> thrust [N]/1
  convert back to double to avoid unexpected data casting/1 -> linear term/1, cmd^2/1

== system exercise03_simulation_model_solution_part1/Reference generator/Signal Builder ==
  Demux : Demux  Tag=STV Demux  Outputs=1
      settings: DisplayOption=none
  FromWs : FromWorkspace  Tag=STV FromWs  VariableName=tuvar
      SigBuilderData=|
      | common.afterFinalStr = 'Extrapolate'
      | common.sampleTime = 0
      | dataSet.timeRange = [0 10]
      | dataSet.name = 'Group 1'
      | sbobj.Groups.Name = 'Group 1'
      | sbobj.Groups.Signals.Name = 'Saw Tooth'
      | sbobj.Groups.Signals.XData = [0 2.5 7.5 10]
      | sbobj.Groups.Signals.YData = [0 1.01 -1 0]
  Saw Tooth : Outport  Tag=STV Outport  VectorParamsAs1DForOutWhenUnconnected=off
  wires:
  Demux/1 -> Saw Tooth/1
  FromWs/1 -> Demux/1

== system exercise03_simulation_model_solution_part1/Controller/inner control loop/convert motor 16-bit command to thrust in Newtons ==
  note: CONVERT MOTOR COMMAND AS uint16 VALUE TO THRUST IN NEWTONS
      | > Apply the following equation:
      | thust [N] = nrotor_vehicle_thrust_max * ( cmd_2_newtons_conversion_quadratic_coefficient * cmd^2 + cmd_2_newtons_conversion_linear_coefficient * cmd )
      |
      | > This sub-system acts element-wise on the input, i.e., the output is a vector of the same length as the input
  cmd [uint16] : Inport
  Add : Sum
  cmd^2 : Math  Operator=square  SignedPower=on
  convert back to double to avoid unexpected data casting : DataTypeConversion  OutDataTypeStr=double  SaturateOnIntegerOverflow=off  RndMeth=Floor
  linear term : Gain  Gain=nrotor_vehicle.thrust_max .* cmd_2_newtons_conversion_linear_coefficient
  quadratic term : Gain  Gain=nrotor_vehicle.thrust_max .* cmd_2_newtons_conversion_quadratic_coefficient
  thrusts [N] : Outport  VectorParamsAs1DForOutWhenUnconnected=off
  wires:
  cmd^2/1 -> quadratic term/1
  quadratic term/1 -> Add/2
  linear term/1 -> Add/1
  cmd [uint16]/1 -> convert back to double to avoid unexpected data casting/1
  Add/1 -> thrusts [N]/1
  convert back to double to avoid unexpected data casting/1 -> linear term/1, cmd^2/1

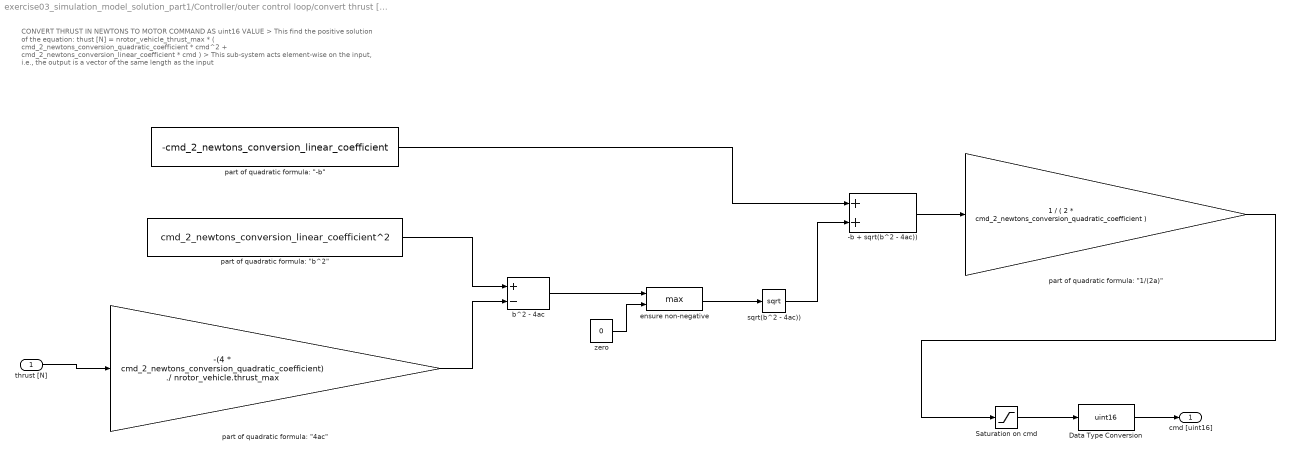
== system exercise03_simulation_model_solution_part1/Controller/outer control loop/convert thrust [N] to [uint16] motor commands ==
  note: CONVERT THRUST IN NEWTONS TO MOTOR COMMAND AS uint16 VALUE
      | > This find the positive solution of the equation:
      | thust [N] = nrotor_vehicle_thrust_max * ( cmd_2_newtons_conversion_quadratic_coefficient * cmd^2 + cmd_2_newtons_conversion_linear_coefficient * cmd )
      |
      | > This sub-system acts element-wise on the input, i.e., the output is a vector of the same length as the input
  thrust [N] : Inport
  -b + sqrt(b^2 - 4ac)) : Sum
  Data Type Conversion : DataTypeConversion  OutDataTypeStr=uint16  SaturateOnIntegerOverflow=off  RndMeth=Floor
  Saturation on cmd : Saturate  UpperLimit=cmd_max  LowerLimit=cmd_min  ZeroCross=off
  b^2 - 4ac : Sum  Inputs=+-
  ensure non-negative : MinMax  Function=max  Inputs=2
  "part of quadratic formula: \"-b\"" : Constant  Value=-cmd_2_newtons_conversion_linear_coefficient
  "part of quadratic formula: \"1/(2a)\"" : Gain  Gain=1 / ( 2 * cmd_2_newtons_conversion_quadratic_coefficient )
  "part of quadratic formula: \"4ac\"" : Gain  Gain=-(4 * cmd_2_newtons_conversion_quadratic_coefficient) ./ nrotor_vehicle.thrust_max
  "part of quadratic formula: \"b^2\"" : Constant  Value=cmd_2_newtons_conversion_linear_coefficient^2
  sqrt(b^2 - 4ac)) : Sqrt
  zero : Constant  Value=0
  cmd [uint16] : Outport  VectorParamsAs1DForOutWhenUnconnected=off
  wires:
  thrust [N]/1 -> "part of quadratic formula: \"4ac\""/1
  Saturation on cmd/1 -> Data Type Conversion/1
  Data Type Conversion/1 -> cmd [uint16]/1
  "part of quadratic formula: \"4ac\""/1 -> b^2 - 4ac/2
  "part of quadratic formula: \"b^2\""/1 -> b^2 - 4ac/1
  b^2 - 4ac/1 -> ensure non-negative/1
  ensure non-negative/1 -> sqrt(b^2 - 4ac))/1
  "part of quadratic formula: \"-b\""/1 -> -b + sqrt(b^2 - 4ac))/1
  sqrt(b^2 - 4ac))/1 -> -b + sqrt(b^2 - 4ac))/2
  -b + sqrt(b^2 - 4ac))/1 -> "part of quadratic formula: \"1/(2a)\""/1
  "part of quadratic formula: \"1/(2a)\""/1 -> Saturation on cmd/1
  zero/1 -> ensure non-negative/2

== matlab function exercise03_simulation_model_solution_part1/Measurements/draw sample from multivariate Gaussian for gyroscope ==
  data: std_normal_rand_sample input; rand_sample output; mean_vector input; covariance_matrix_decomposition input
function rand_sample = mvn_gyroscope( std_normal_rand_sample , mean_vector , covariance_matrix_decomposition )


% Compute the multi-variate Gaussian sample from a distirbution with:
% > "mean_vector" as the mean, and
% > "covariance_matrix_decomposition" as the "square root" of the
%    covariance matrix
rand_sample = mean_vector + covariance_matrix_decomposition * std_normal_rand_sample;

== matlab function exercise03_simulation_model_solution_part1/Measurements/draw sample from multivariate Gaussian for full state ==
  data: std_normal_rand_sample input; rand_sample output; mean_vector input; covariance_matrix_decomposition input
function rand_sample = mvn_full_state( std_normal_rand_sample , mean_vector , covariance_matrix_decomposition )


% Compute the multi-variate Gaussian sample from a distirbution with:
% > "mean_vector" as the mean, and
% > "covariance_matrix_decomposition" as the "square root" of the
%    covariance matrix
rand_sample = mean_vector + covariance_matrix_decomposition * std_normal_rand_sample;

== matlab function exercise03_simulation_model_solution_part1/Measurements/draw sample from multivariate Gaussian for accelerometer ==
  data: std_normal_rand_sample input; rand_sample output; mean_vector input; covariance_matrix_decomposition input
function rand_sample = mvn_accelerometer( std_normal_rand_sample , mean_vector , covariance_matrix_decomposition )


% Compute the multi-variate Gaussian sample from a distirbution with:
% > "mean_vector" as the mean, and
% > "covariance_matrix_decomposition" as the "square root" of the
%    covariance matrix
rand_sample = mean_vector + covariance_matrix_decomposition * std_normal_rand_sample;

== matlab function exercise03_simulation_model_solution_part1/Controller/inner control loop/compute the per-propeller thrust desired ==
  data: cmd_per_motor_desired input; cmd_for_body_torques_desired input; cmd_to_apply output
function cmd_to_apply = distribute_power( cmd_per_motor_desired , cmd_for_body_torques_desired )
% ----------------------------------------------------------------------- %
% DESCRIPTION:
% This function computes the uint16 command to apply to each motor as per
% the code that runs "on-board" on the Crazyflie's firmware
%
%
% INPUT ARGUMENTS:
%
% cmd_per_motor_desired [uint16]
% > This is a colulmn vector with length equal to the number of propellers
%   on the Crazyflie, i.e., 4, and each element represents the "baseline"
%   16-bit command that should be requested from the Crazyflie, as
%   requested by the outer loop controller.
%
% cmd_for_body_torques_desired [uint16]
% > This is the "actuation" uint16 command that comes directly from the
%   output of the Crazyflie's body rate PID controllers running in the
%   firmware. This value of command has already been adjust for the
%   dimensions of the Crazyflie, and the pattern for distributing the
%   command across the motor is provided in the exercise sheet.
%
%
% RETURN ARGUMENTS:
% % cmd_to_apply [uint16]
% > This is a colulmn vector with length equal to the number of propellers
%   on the Crazyflie, i.e., 4, and each element represents the 16-bit
%   command that will be requested from the motors
%
%
% DATA FORMAT ASSUMPTIONS:
% > the "cmd_per_motor_desired" vector is such when applied, the static
%   thrusts exert no torque about the body frame axes
%
% ----------------------------------------------------------------------- %


% Get the uint16 commands into a separate variable for each motor
cmd1 = cmd_per_motor_desired(1);
cmd2 = cmd_per_motor_desired(2);
cmd3 = cmd_per_motor_desired(3);
cmd4 = cmd_per_motor_desired(4);


% Get the desired body torques uint16 commands into a separate variable for
% the "uint16 command torque" desired about each of the body frame axes
r = cmd_for_body_torques_desired(1) / 2;
p = cmd_for_body_torques_desired(2) / 2;
y = cmd_for_body_torques_desired(3);


% These variable names have been used to partially match the code from the
% Crazyflie firmware:
% r  -  where "r" stands for roll, this is the "uint16 command torque" to
%       apply about the body-frame's x-axis, i.e., the roll-axis
% p  -  where "p" stands for pitch, this is the "uint16 command torque" to
%       apply about the body-frame's y-axis, i.e., the pitch-axis
% y  -  where "y" stands for yaw, this is the "uint16 command torque" to
%       apply about the body-frame's z-axis, i.e., the yaw-axis
%
% Note: the "/ 2" for the extraction of "r" and "p" above is simply added
% to minimic the code of the Crazyflie firmware. Presumably the Crazyflie's
% PID contollers for the body-frame roll and pitch axis are tuned with this
% factor of "/ 2" appropriately accounted for.


% Initialise the return variable "cmd_to_apply" to zeros
% > This can be required so that Simulink knows the expected size
cmd_to_apply = zeros(4,1);

% Compute the 16-bit command that should be applied from each motor as per
% the code from the Crazyflie firmware
% > For motor 1:
cmd_to_apply(1,1)  =  cmd1   - r   + p  +  y;
% > For motor 1:
cmd_to_apply(2,1)  =  cmd2   - r   - p  -  y;
% > For motor 1:
cmd_to_apply(3,1)  =  cmd3   + r   - p  +  y;
% > For motor 1:
cmd_to_apply(4,1)  =  cmd4   + r   + p  -  y;
